simulink model "Stateflow_Model_test"  (R2013b)
settings: Solver=ode45  StartTime=0.0  StopTime=10.0  RelTol=1e-3
settings Model: Creator=daltdoer  LastModifiedBy=daltdoer

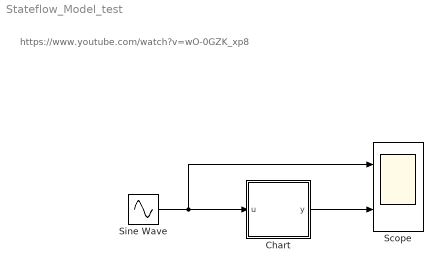
== system Stateflow_Model_test ==
  note: https://www.youtube.com/watch?v=wO-0GZK_xp8
  Chart : Stateflow chart  TreatAsAtomicUnit=on
  Scope : Scope  NumInputPorts=2
      settings: YMin=-5~-5  YMax=5~5
  Sine Wave : Sin  SampleTime=0
  wires:
  Sine Wave/1 -> Chart/1(u), Scope/1
  Chart/1(y) -> Scope/2

== stateflow chart Stateflow_Model_test/Chart ==
  state ON
    y = 1;
  state OFF
    y = -1;
  (default) -> ON
  ON -> OFF : [u<0]
  OFF -> ON : [u>0]
  data: u input; y output double
